simulink model "circle_sim"  (R2021b)
settings: Solver=ode4  StartTime=0.0  StopTime=5  FixedStep=Ts  RelTol=1e-3  EnableMultiTasking=on
undefined symbols (not defined in the file or in its folder): q0, q0dot
settings Model: Creator=giusepp  LastModifiedBy=Rita
settings SolverCC: AlgebraicLoopSolver=TrustRegion
settings DataIOCC: LimitDataPoints=on  SaveFormat=Array  ReturnWorkspaceOutputs=off
settings OptimizationCC: LifeSpan=inf
settings DebuggingCC: SolverPrmCheckMsg=warning  SFUnexpectedBacktrackingDiag=warning  SFNoUnconditionalDefaultTransitionDiag=warning  SFExecutionAtInitializationDiag=none  SFMachineParentedDataDiag=warning  ArithmeticOperatorsInVariantConditions=warning
settings HardwareCC: ProdBitPerPointer=32  ProdBitPerSizeT=32  ProdBitPerPtrDiffT=32  ProdLargestAtomicFloat=None  ProdIntDivRoundTo=Undefined  ProdEndianess=Unspecified  ProdWordSize=32  ProdHWDeviceType=32-bit Generic
settings ModelReferenceCC: PropagateSignalLabelsOutOfModel=off
settings SFSimCC: SimUseLocalCustomCode=off  CustomCodeUndefinedFunction=UseInterfaceOnly
settings RTWCC: RTWUseLocalCustomCode=off
settings CodeAppCC: StateflowObjectComments=on
settings GRTTargetCC: TargetLangStandard=C89/C90 (ANSI)
settings ConfigComp: CovMetricSettings=dw  CovSaveCumulativeToWorkspaceVar=on  CovSaveSingleToWorkspaceVar=on  CovExternalEMLEnable=off  CovSFcnEnable=off

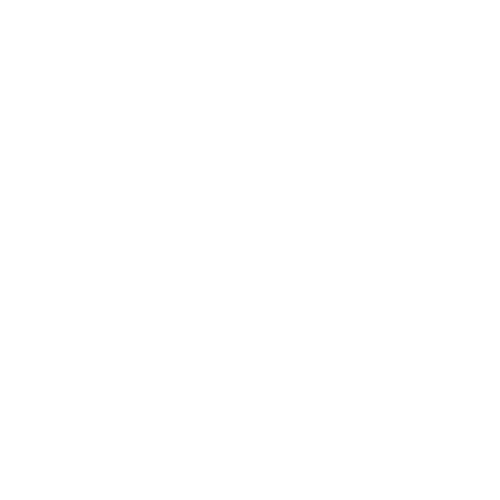
[thumbnail: Simulink's stored preview of the top-level diagram]
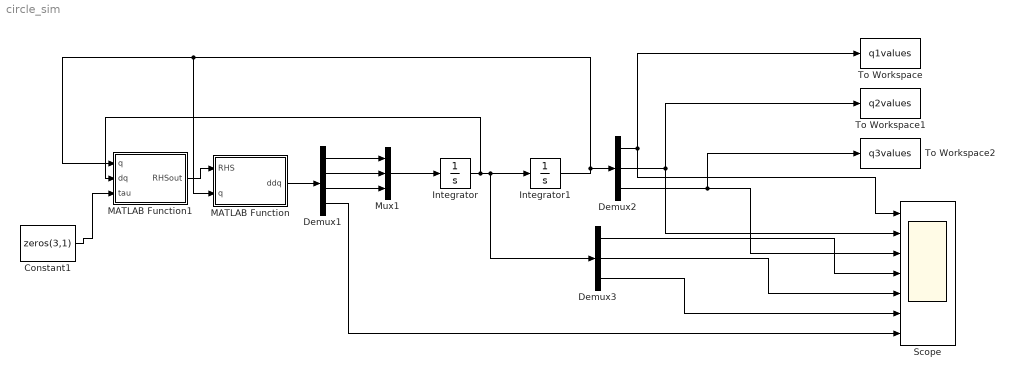
== system circle_sim ==
  Constant1 : Constant  Value=zeros(3,1)
  Demux1 : Demux
  Demux2 : Demux  Outputs=3
  Demux3 : Demux  Outputs=3
  Integrator : Integrator  InitialCondition=q0dot
  Integrator1 : Integrator  InitialCondition=q0
  MATLAB Function : MATLAB Function  TreatAsAtomicUnit=on
  MATLAB Function1 : MATLAB Function  TreatAsAtomicUnit=on
  Mux1 : Mux  Inputs=3
  Scope : Scope  NumInputPorts=7
  To Workspace : ToWorkspace  VariableName=q1values  SaveFormat=Timeseries  SampleTime=-1
  To Workspace1 : ToWorkspace  VariableName=q2values  SaveFormat=Timeseries  SampleTime=-1
  To Workspace2 : ToWorkspace  VariableName=q3values  SaveFormat=Timeseries  SampleTime=-1
  wires:
  Integrator/1 -> Demux3/1, Integrator1/1, MATLAB Function1/2(dq)
  Integrator1/1 -> MATLAB Function1/1(q), MATLAB Function/2(q), Demux2/1
  Demux2/1 -> Scope/1, To Workspace/1
  Demux2/2 -> Scope/2, To Workspace1/1
  Demux3/1 -> Scope/4
  Demux3/2 -> Scope/5
  MATLAB Function/1(ddq) -> Demux1/1
  Demux1/1 -> Mux1/1
  Demux1/2 -> Mux1/2
  Mux1/1 -> Integrator/1
  MATLAB Function1/1(RHSout) -> MATLAB Function/1(RHS)
  Constant1/1 -> MATLAB Function1/3(tau)
  Demux1/4 -> Scope/7
  Demux1/3 -> Mux1/3
  Demux3/3 -> Scope/6
  Demux2/3 -> To Workspace2/1, Scope/3

== matlab function circle_sim/MATLAB Function ==
  data: RHS input; q input; ddq output
function ddq = MassMatrix(RHS,q)

IM = modifiedInertiaMatrix(q);

ddq = IM\RHS;

== matlab function circle_sim/MATLAB Function1 ==
  data: q input; RHSout output; dq input; tau input
function RHSout = fcn(q,dq,tau)

RHSout = RHS(q,dq,tau);
